simulink model "verify_Xue_block"  (R2018a)
settings: Solver=ode4  StartTime=0.0  StopTime=10.0  FixedStep=0.01  RelTol=1e-3
settings Model: Creator=lenovo  LastModifiedBy=standard

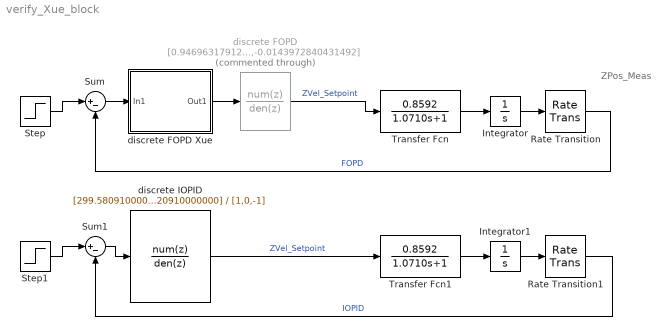
== system verify_Xue_block ==
  note: ZPos_Meas
  Integrator : Integrator
  Integrator1 : Integrator
  Rate Transition : RateTransition  OutPortSampleTime=0.01
  Rate Transition1 : RateTransition  OutPortSampleTime=0.01
  Step : Step  SampleTime=0.01
  Step1 : Step  SampleTime=0.01
  Sum : Sum  Inputs=|+-
  Sum1 : Sum  Inputs=|+-
  Transfer Fcn : TransferFcn  Numerator=[0.8592]  Denominator=[1.0710 1]
  Transfer Fcn1 : TransferFcn  Numerator=[0.8592]  Denominator=[1.0710 1]
  discrete FOPD : DiscreteTransferFcn  Commented=through  Numerator=[0.946963179122833,-2.77792961698899,2.98392102212133,-1.40760552266944,0.267978964388861,-0.0129932830769816]  Denominator=[1,-2.94510699389959,3.17934233429781,-1.51000556757338,0.290497513211450,-0.0143972840431492]  SampleTime=0.01
  discrete FOPD Xue : Subsystem
  discrete IOPID : DiscreteTransferFcn  Numerator=[299.580910000000,-595.998180000000,296.420910000000]  Denominator=[1,0,-1]  SampleTime=0.01
  wires:
  Step/1 -> Sum/1
  discrete FOPD/1 -> Transfer Fcn/1  "ZVel_Setpoint"
  Transfer Fcn/1 -> Integrator/1
  Integrator/1 -> Rate Transition/1
  Rate Transition/1 -> Sum/2  "FOPD"
  Step1/1 -> Sum1/1
  discrete IOPID/1 -> Transfer Fcn1/1  "ZVel_Setpoint"
  Sum1/1 -> discrete IOPID/1
  Transfer Fcn1/1 -> Integrator1/1
  Rate Transition1/1 -> Sum1/2  "IOPID"
  Integrator1/1 -> Rate Transition1/1
  Sum/1 -> discrete FOPD Xue/1(In1)
  discrete FOPD Xue/1(Out1) -> discrete FOPD/1

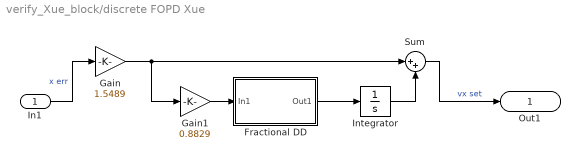
== system verify_Xue_block/discrete FOPD Xue ==
  In1 : Inport
  Fractional DD : Subsystem  mask{gam=1.9885, ww=[1e-3, 1e3], n=5, kF1=on, kF=Modified Oustaloup filter}
      mask prompts: gam "Derivative order gamma"; ww "Frequency range [wb,wh]"; n "Apprixmation order"; kF1 "Is a low-pass filter required?"; kF "Filter type"
      mask init:
      | wb=ww(1); wh=ww(2); 
      | if kF==1, G=ousta_fod(gam,n,wb,wh);
      | else, G=new_fod(gam,n,wb,wh); end
      | num=G.num{1}; den=G.den{1}; T=1/wh; str='Fractional\n';
      | if isnumeric(gam)
      | 	if gam>0, str=[str, 'Der  s^' num2str(gam) ];
      | 	else, str=[str, 'Int  s^{' num2str(gam) '}']; end
      | else, str=[str, 'Der  s^gam']; end
      | if kF1==1, G=G*tf(1,[T 1]); end
      mask TypeOptions kF: Oustaloup filter | Modified Oustaloup filter | Matsuda-Fujii filter
      mask Display: disp(str)
  Gain : Gain  Gain=1.5489
  Gain1 : Gain  Gain=0.8829
  Integrator : Integrator
  Sum : Sum  Inputs=|++
  Out1 : Outport
  wires:
  Sum/1 -> Out1/1  "vx set"
  In1/1 -> Gain/1  "x err"
  Gain/1 -> Gain1/1, Sum/1
  Fractional DD/1(Out1) -> Integrator/1
  Gain1/1 -> Fractional DD/1(In1)
  Integrator/1 -> Sum/2

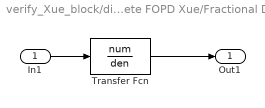
== system verify_Xue_block/discrete FOPD Xue/Fractional DD ==
  In1 : Inport
  Transfer Fcn : TransferFcn  Numerator=num  Denominator=den
  Out1 : Outport
  wires:
  Transfer Fcn/1 -> Out1/1
  In1/1 -> Transfer Fcn/1
